simulink model "S1_ContinuousDCMotorSimulationSampled"  (R2018b)
settings: Solver=VariableStepAuto  StartTime=0.0  StopTime=25  MaxStep=Ts  RelTol=1e-3
undefined symbols (not defined in the file): C0, DiscIntNeverNeededParam, F, Imax, Imin, J, Ke, Km, Kphi, L, R, Ts, TsMeca, Vmax, Vmin
libraries: simulink x7
Description:
  | Continuous time model of the DC motor
  | 
  | Cascaded speed control :
  | - Inner loop : electrical control (state feedback with integral action)
  | - Outer loop :  mechanical control (state feedback with integral action)
  | - Clamping : Enable or disable integral actions
settings Model: Creator=R.Delpoux & L.Kerhuel  LastModifiedBy=rdelpoux
settings SolverCC: ZeroCrossControl=DisableAll
settings SFSimCC: SimUseLocalCustomCode=off
settings RTWCC: RTWUseLocalCustomCode=off

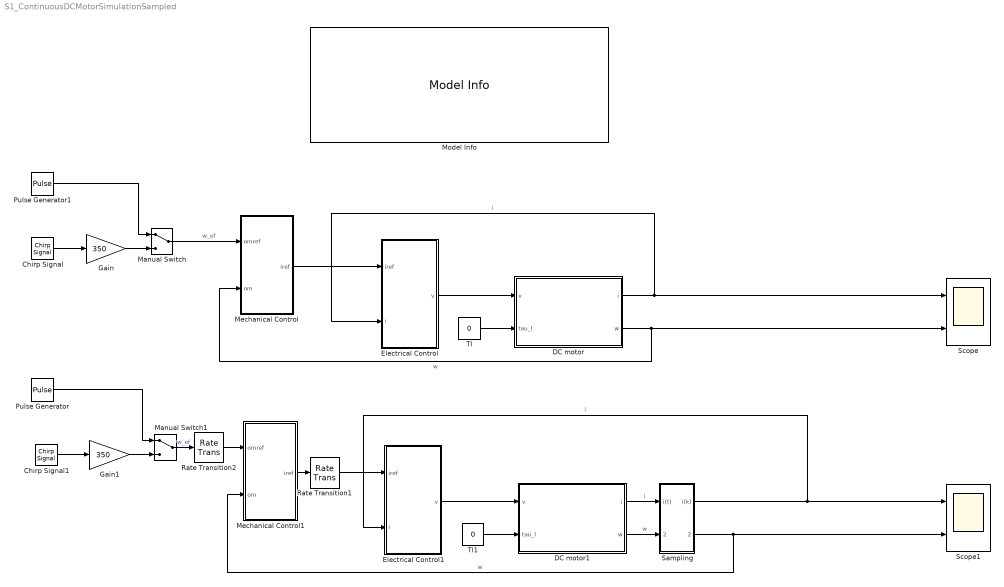
== system S1_ContinuousDCMotorSimulationSampled ==
  Chirp Signal : simulink/Sources/Chirp Signal  f1=0.1  T=20  f2=5
  Chirp Signal1 : simulink/Sources/Chirp Signal  f1=0.1  T=20  f2=5
  DC motor : Subsystem  mask(Motor PRAVALUX MPM4-0002){R=R, L=L, Kphi=Kphi, J=J, F=F, C0=C0}
      mask prompts: R "Resistance (R) in Ohms"; L "Inductance (L) in H"; Kphi "Back EMF (Kphi) in V/rad/s"; J "J in kgm²"; F "F in N/rad/s"
      mask help:
      | Continuous time Model for PRAVALUX MPM4 DC motor
      | Caracteristics: 24V DC, 90W, 5.2A, 3000RPM
      |
      | It is a 2nd order model made of two intertwinned system:
      | one 1st order electrical system and one 1st order mechanical system.
      |
      | Look under mask (Ctrl-U) to see the model
      mask DialogControl Container11 Prompt: Motor
      mask DialogControl Container3 Prompt: Electrical Parameters
      mask DialogControl Container3_copy Prompt: Mechanical Parameters
      mask Display:
      | color('green');
      | image('MotorPravalux.png');
      | %port_label('input',1,'DC');
      | %port_label('output',1,'BEMF');
  DC motor1 : Subsystem  mask(Motor PRAVALUX MPM4-0002){R=R, L=L, Kphi=Kphi, J=J, F=F, C0=C0}
      mask prompts: R "Resistance (R) in Ohms"; L "Inductance (L) in H"; Kphi "Back EMF (Kphi) in V/rad/s"; J "J in kgm²"; F "F in N/rad/s"
      mask help:
      | Continuous time Model for PRAVALUX MPM4 DC motor
      | Caracteristics: 24V DC, 90W, 5.2A, 3000RPM
      |
      | It is a 2nd order model made of two intertwinned system:
      | one 1st order electrical system and one 1st order mechanical system.
      |
      | Look under mask (Ctrl-U) to see the model
      mask DialogControl Container11 Prompt: Motor
      mask DialogControl Container3 Prompt: Electrical Parameters
      mask DialogControl Container3_copy Prompt: Mechanical Parameters
      mask Display:
      | color('green');
      | image('MotorPravalux.png');
      | %port_label('input',1,'DC');
      | %port_label('output',1,'BEMF');
  Electrical Control : Subsystem
  Electrical Control1 : Subsystem
  Gain : Gain  Gain=350  OutDataTypeStr=Inherit: Inherit via back propagation
  Gain1 : Gain  Gain=350  OutDataTypeStr=Inherit: Inherit via back propagation
  Manual Switch : ManualSwitch
  Manual Switch1 : ManualSwitch
  Mechanical Control : Subsystem
  Mechanical Control1 : Subsystem
  Model Info : simulink/Model-Wide Utilities/Model Info  Frame=on  DisplayStringWithTags=|  HorizontalTextAlignment=Center  LeftAlignmentValue=0.5
      | %<ModelName> v%<ModelVersion> - %<Creator>
      | 
      | %<Description>
      | 
      | Lost modified on: %<LastModificationDate>
  Pulse Generator : DiscretePulseGenerator  PulseType=Time based  Amplitude=200  PulseWidth=50  PhaseDelay=0.5  SampleTime=-1
  Pulse Generator1 : DiscretePulseGenerator  PulseType=Time based  Amplitude=200  PulseWidth=50  PhaseDelay=0.5  SampleTime=-1
  Rate Transition1 : RateTransition  Deterministic=off
  Rate Transition2 : RateTransition  Deterministic=off
  Sampling : Subsystem
  Scope : Scope  NumInputPorts=2
  Scope1 : Scope  NumInputPorts=2
  Tl : Constant  Value=0
  Tl1 : Constant  Value=0
  wires:
  Electrical Control/1(v) -> DC motor/1(v)
  DC motor/1(i) -> Electrical Control/2(i), Scope/1  "i"
  DC motor/2(w) -> Scope/2, Mechanical Control/2(om)  "w"
  Manual Switch/1 -> Mechanical Control/1(omref)  "w_ef"
  Mechanical Control/1(iref) -> Electrical Control/1(iref)
  Tl/1 -> DC motor/2(tau_l)
  Gain/1 -> Manual Switch/2
  Chirp Signal/1 -> Gain/1
  Pulse Generator1/1 -> Manual Switch/1
  Pulse Generator/1 -> Manual Switch1/1
  Electrical Control1/1(v) -> DC motor1/1(v)
  Tl1/1 -> DC motor1/2(tau_l)
  Gain1/1 -> Manual Switch1/2
  Chirp Signal1/1 -> Gain1/1
  Manual Switch1/1 -> Rate Transition2/1  "w_ef"
  DC motor1/1(i) -> Sampling/1(i(t))  "i"
  DC motor1/2(w) -> Sampling/2(w(t))  "w"
  Sampling/1(i(k)) -> Electrical Control1/2(i), Scope1/1  "i"
  Sampling/2(w(k)) -> Scope1/2, Mechanical Control1/2(om)  "w"
  Mechanical Control1/1(iref) -> Rate Transition1/1
  Rate Transition1/1 -> Electrical Control1/1(iref)
  Rate Transition2/1 -> Mechanical Control1/1(omref)

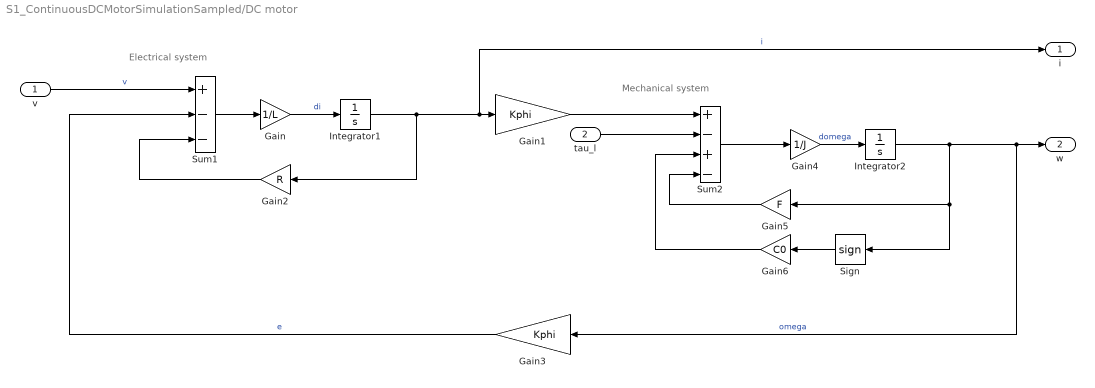
== system S1_ContinuousDCMotorSimulationSampled/DC motor ==
  note: Mechanical system
  note: Electrical system
  v : Inport  SampleTime=0
  tau_l : Inport  Port=2
  Gain : Gain  Gain=1/L
  Gain1 : Gain  Gain=Kphi
  Gain2 : Gain  Gain=R
  "Gain3  " : Gain  Gain=Kphi
  Gain4 : Gain  Gain=1/J
  Gain5 : Gain  Gain=F
  Gain6 : Gain  Gain=C0
  Integrator1 : Integrator
  Integrator2 : Integrator
  Sign : Signum
  Sum1 : Sum  Inputs=+--
  Sum2 : Sum  Inputs=+-+-
  i : Outport
  w : Outport  Port=2
  wires:
  Sum1/1 -> Gain/1
  Gain/1 -> Integrator1/1  "di"
  Integrator1/1 -> Gain2/1, i/1, Gain1/1  "i"
  v/1 -> Sum1/1  "v"
  Gain2/1 -> Sum1/3
  "Gain3  "/1 -> Sum1/2  "e"
  tau_l/1 -> Sum2/2
  Gain6/1 -> Sum2/3
  Sign/1 -> Gain6/1
  Integrator2/1 -> "Gain3  "/1, w/1, Sign/1, Gain5/1  "omega"
  Gain5/1 -> Sum2/4
  Sum2/1 -> Gain4/1
  Gain4/1 -> Integrator2/1  "domega"
  Gain1/1 -> Sum2/1

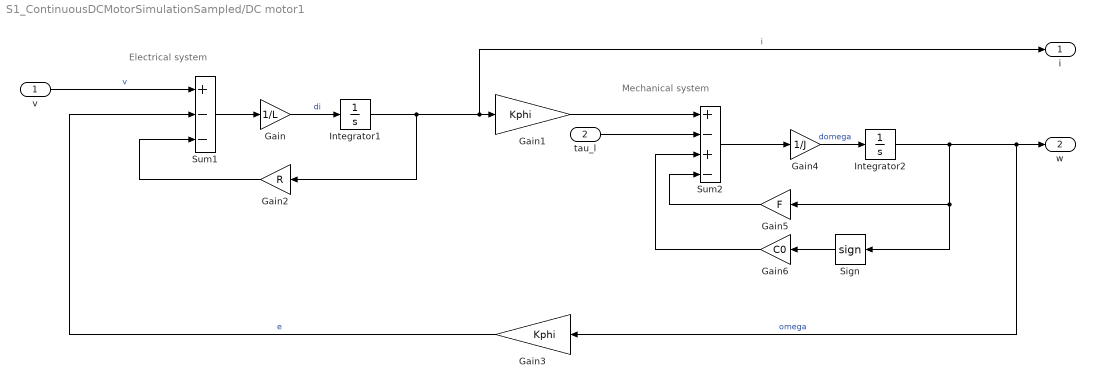
== system S1_ContinuousDCMotorSimulationSampled/DC motor1 ==
  note: Mechanical system
  note: Electrical system
  v : Inport  SampleTime=0
  tau_l : Inport  Port=2
  Gain : Gain  Gain=1/L
  Gain1 : Gain  Gain=Kphi
  Gain2 : Gain  Gain=R
  "Gain3  " : Gain  Gain=Kphi
  Gain4 : Gain  Gain=1/J
  Gain5 : Gain  Gain=F
  Gain6 : Gain  Gain=C0
  Integrator1 : Integrator
  Integrator2 : Integrator
  Sign : Signum
  Sum1 : Sum  Inputs=+--
  Sum2 : Sum  Inputs=+-+-
  i : Outport
  w : Outport  Port=2
  wires:
  Sum1/1 -> Gain/1
  Gain/1 -> Integrator1/1  "di"
  Integrator1/1 -> Gain2/1, i/1, Gain1/1  "i"
  v/1 -> Sum1/1  "v"
  Gain2/1 -> Sum1/3
  "Gain3  "/1 -> Sum1/2  "e"
  tau_l/1 -> Sum2/2
  Gain6/1 -> Sum2/3
  Sign/1 -> Gain6/1
  Integrator2/1 -> "Gain3  "/1, w/1, Sign/1, Gain5/1  "omega"
  Gain5/1 -> Sum2/4
  Sum2/1 -> Gain4/1
  Gain4/1 -> Integrator2/1  "domega"
  Gain1/1 -> Sum2/1

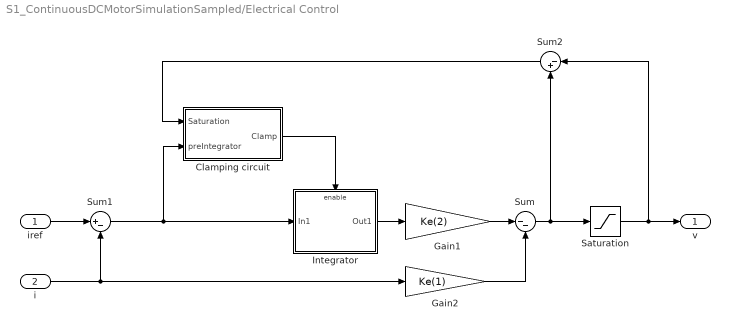
== system S1_ContinuousDCMotorSimulationSampled/Electrical Control ==
  iref : Inport
  i : Inport  Port=2
  Clamping circuit : Subsystem
  Gain1 : Gain  Gain=Ke(2)
  Gain2 : Gain  Gain=Ke(1)
  Integrator : Subsystem
  Saturation : Saturate  UpperLimit=Vmax  LowerLimit=Vmin
  Sum : Sum  Inputs=|--
  Sum1 : Sum  Inputs=|+-
  Sum2 : Sum  Inputs=|-+  OutDataTypeStr=Inherit: Same as accumulator
  v : Outport
  wires:
  iref/1 -> Sum1/1
  i/1 -> Gain2/1, Sum1/2
  Gain1/1 -> Sum/1
  Gain2/1 -> Sum/2
  Saturation/1 -> Sum2/1, v/1
  Sum1/1 -> Integrator/1(In1), Clamping circuit/2(preIntegrator)
  Integrator/1(Out1) -> Gain1/1
  Clamping circuit/1(Clamp) -> Integrator/Enable
  Sum/1 -> Saturation/1, Sum2/2
  Sum2/1 -> Clamping circuit/1(Saturation)

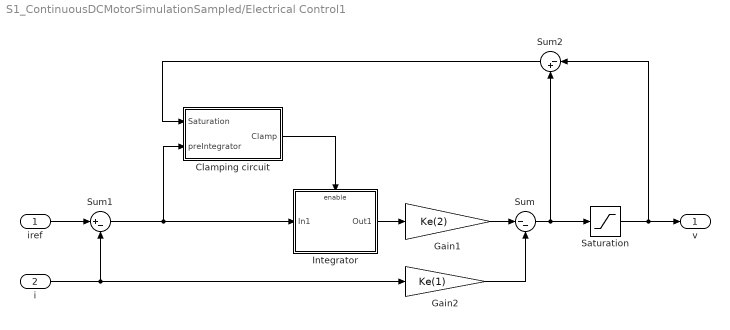
== system S1_ContinuousDCMotorSimulationSampled/Electrical Control1 ==
  iref : Inport
  i : Inport  Port=2
  Clamping circuit : Subsystem
  Gain1 : Gain  Gain=Ke(2)
  Gain2 : Gain  Gain=Ke(1)
  Integrator : Subsystem
  Saturation : Saturate  UpperLimit=Vmax  LowerLimit=Vmin
  Sum : Sum  Inputs=|--
  Sum1 : Sum  Inputs=|+-
  Sum2 : Sum  Inputs=|-+  OutDataTypeStr=Inherit: Same as accumulator
  v : Outport
  wires:
  iref/1 -> Sum1/1
  i/1 -> Gain2/1, Sum1/2
  Gain1/1 -> Sum/1
  Gain2/1 -> Sum/2
  Saturation/1 -> Sum2/1, v/1
  Sum1/1 -> Integrator/1(In1), Clamping circuit/2(preIntegrator)
  Integrator/1(Out1) -> Gain1/1
  Clamping circuit/1(Clamp) -> Integrator/Enable
  Sum/1 -> Saturation/1, Sum2/2
  Sum2/1 -> Clamping circuit/1(Saturation)

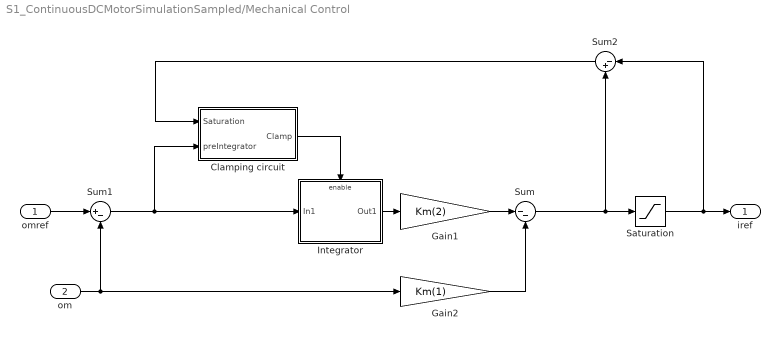
== system S1_ContinuousDCMotorSimulationSampled/Mechanical Control ==
  omref : Inport
  om : Inport  Port=2
  Clamping circuit : Subsystem
  Gain1 : Gain  Gain=Km(2)
  Gain2 : Gain  Gain=Km(1)
  Integrator : Subsystem
  Saturation : Saturate  UpperLimit=Imax  LowerLimit=Imin
  Sum : Sum  Inputs=|--
  Sum1 : Sum  Inputs=|+-
  Sum2 : Sum  Inputs=|-+  OutDataTypeStr=Inherit: Same as accumulator
  iref : Outport
  wires:
  Gain1/1 -> Sum/1
  Sum1/1 -> Clamping circuit/2(preIntegrator), Integrator/1(In1)
  omref/1 -> Sum1/1
  Gain2/1 -> Sum/2
  om/1 -> Gain2/1, Sum1/2
  Sum2/1 -> Clamping circuit/1(Saturation)
  Sum/1 -> Sum2/2, Saturation/1
  Clamping circuit/1(Clamp) -> Integrator/Enable
  Saturation/1 -> Sum2/1, iref/1
  Integrator/1(Out1) -> Gain1/1

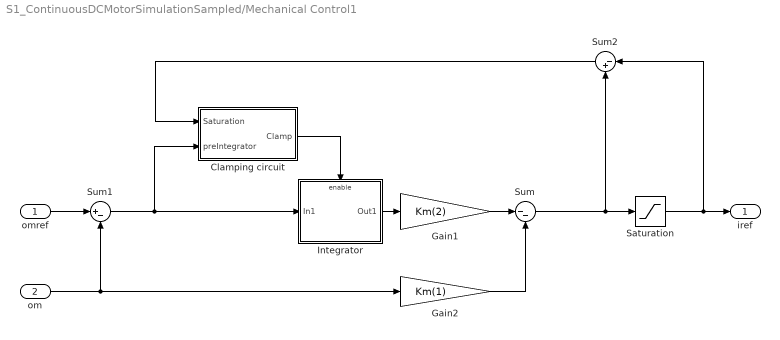
== system S1_ContinuousDCMotorSimulationSampled/Mechanical Control1 ==
  omref : Inport
  om : Inport  Port=2
  Clamping circuit : Subsystem
  Gain1 : Gain  Gain=Km(2)
  Gain2 : Gain  Gain=Km(1)
  Integrator : Subsystem
  Saturation : Saturate  UpperLimit=Imax  LowerLimit=Imin
  Sum : Sum  Inputs=|--
  Sum1 : Sum  Inputs=|+-
  Sum2 : Sum  Inputs=|-+  OutDataTypeStr=Inherit: Same as accumulator
  iref : Outport
  wires:
  Gain1/1 -> Sum/1
  Sum1/1 -> Clamping circuit/2(preIntegrator), Integrator/1(In1)
  omref/1 -> Sum1/1
  Gain2/1 -> Sum/2
  om/1 -> Gain2/1, Sum1/2
  Sum2/1 -> Clamping circuit/1(Saturation)
  Sum/1 -> Sum2/2, Saturation/1
  Clamping circuit/1(Clamp) -> Integrator/Enable
  Saturation/1 -> Sum2/1, iref/1
  Integrator/1(Out1) -> Gain1/1

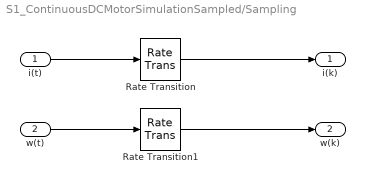
== system S1_ContinuousDCMotorSimulationSampled/Sampling ==
  i(t) : Inport
  w(t) : Inport  Port=2
  Rate Transition : RateTransition  Deterministic=off  OutPortSampleTime=Ts
  Rate Transition1 : RateTransition  Deterministic=off  OutPortSampleTime=TsMeca
  i(k) : Outport
  w(k) : Outport  Port=2
  wires:
  Rate Transition/1 -> i(k)/1
  i(t)/1 -> Rate Transition/1
  w(t)/1 -> Rate Transition1/1
  Rate Transition1/1 -> w(k)/1

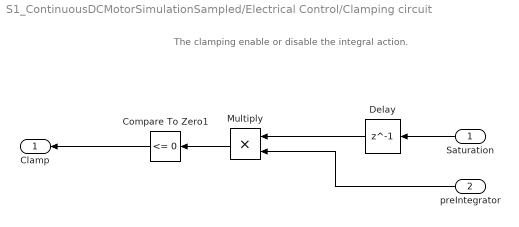
== system S1_ContinuousDCMotorSimulationSampled/Electrical Control/Clamping circuit ==
  note: The clamping enable or disable the integral action.
  Saturation : Inport  DisableCoverage=on
  preIntegrator : Inport  DisableCoverage=on  Port=2
  Compare To Zero1 : simulink/Logic and Bit Operations/Compare To Zero  relop=<=  OutDataTypeStr=boolean
  Delay : Delay  DelayLength=1  InitialCondition=0
  Multiply : Product
  Clamp : Outport  DisableCoverage=on
  wires:
  Compare To Zero1/1 -> Clamp/1
  preIntegrator/1 -> Multiply/2
  Multiply/1 -> Compare To Zero1/1
  Saturation/1 -> Delay/1
  Delay/1 -> Multiply/1

== system S1_ContinuousDCMotorSimulationSampled/Electrical Control/Integrator ==
  In1 : Inport
  Enable : EnablePort
  Integrator : Integrator
  Out1 : Outport
  wires:
  Integrator/1 -> Out1/1
  In1/1 -> Integrator/1

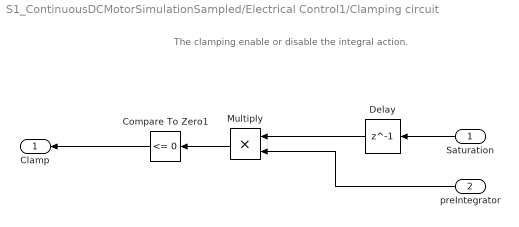
== system S1_ContinuousDCMotorSimulationSampled/Electrical Control1/Clamping circuit ==
  note: The clamping enable or disable the integral action.
  Saturation : Inport  DisableCoverage=on
  preIntegrator : Inport  DisableCoverage=on  Port=2
  Compare To Zero1 : simulink/Logic and Bit Operations/Compare To Zero  relop=<=  OutDataTypeStr=boolean
  Delay : Delay  DelayLength=1  InitialCondition=0
  Multiply : Product
  Clamp : Outport  DisableCoverage=on
  wires:
  Compare To Zero1/1 -> Clamp/1
  preIntegrator/1 -> Multiply/2
  Multiply/1 -> Compare To Zero1/1
  Saturation/1 -> Delay/1
  Delay/1 -> Multiply/1

== system S1_ContinuousDCMotorSimulationSampled/Electrical Control1/Integrator ==
  In1 : Inport
  Enable : EnablePort
  Discrete-Time Integrator : DiscreteIntegrator  SampleTime=Ts  ICPrevOutput=DiscIntNeverNeededParam  ICPrevScaledInput=DiscIntNeverNeededParam
  Out1 : Outport
  wires:
  Discrete-Time Integrator/1 -> Out1/1
  In1/1 -> Discrete-Time Integrator/1

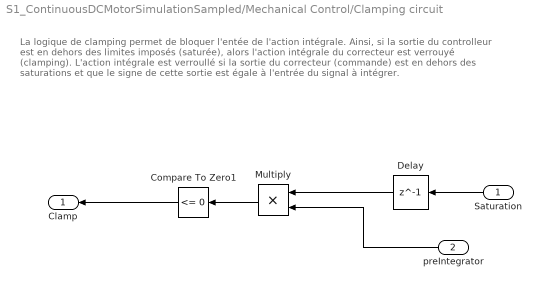
== system S1_ContinuousDCMotorSimulationSampled/Mechanical Control/Clamping circuit ==
  note: La logique de clamping permet de bloquer l'entée de l'action intégrale.
      | Ainsi, si la sortie du controlleur est en dehors des limites imposés (saturée), alors l'action intégrale du correcteur est verrouyé (clamping).
      | L'action intégrale est verroullé si la sortie du correcteur (commande) est en dehors des saturations et que le signe de cette sortie est égale
      | à l'entrée du signal à intégrer.
  Saturation : Inport  DisableCoverage=on
  preIntegrator : Inport  DisableCoverage=on  Port=2
  Compare To Zero1 : simulink/Logic and Bit Operations/Compare To Zero  relop=<=  OutDataTypeStr=boolean
  Delay : Delay  DelayLength=1  InitialCondition=0
  Multiply : Product
  Clamp : Outport  DisableCoverage=on
  wires:
  Compare To Zero1/1 -> Clamp/1
  preIntegrator/1 -> Multiply/2
  Multiply/1 -> Compare To Zero1/1
  Saturation/1 -> Delay/1
  Delay/1 -> Multiply/1

== system S1_ContinuousDCMotorSimulationSampled/Mechanical Control/Integrator ==
  In1 : Inport
  Enable : EnablePort
  Integrator : Integrator
  Out1 : Outport
  wires:
  Integrator/1 -> Out1/1
  In1/1 -> Integrator/1

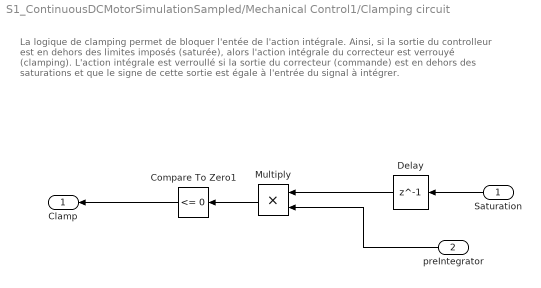
== system S1_ContinuousDCMotorSimulationSampled/Mechanical Control1/Clamping circuit ==
  note: La logique de clamping permet de bloquer l'entée de l'action intégrale.
      | Ainsi, si la sortie du controlleur est en dehors des limites imposés (saturée), alors l'action intégrale du correcteur est verrouyé (clamping).
      | L'action intégrale est verroullé si la sortie du correcteur (commande) est en dehors des saturations et que le signe de cette sortie est égale
      | à l'entrée du signal à intégrer.
  Saturation : Inport  DisableCoverage=on
  preIntegrator : Inport  DisableCoverage=on  Port=2
  Compare To Zero1 : simulink/Logic and Bit Operations/Compare To Zero  relop=<=  OutDataTypeStr=boolean
  Delay : Delay  DelayLength=1  InitialCondition=0
  Multiply : Product
  Clamp : Outport  DisableCoverage=on
  wires:
  Compare To Zero1/1 -> Clamp/1
  preIntegrator/1 -> Multiply/2
  Multiply/1 -> Compare To Zero1/1
  Saturation/1 -> Delay/1
  Delay/1 -> Multiply/1

== system S1_ContinuousDCMotorSimulationSampled/Mechanical Control1/Integrator ==
  In1 : Inport
  Enable : EnablePort
  Discrete-Time Integrator : DiscreteIntegrator  SampleTime=TsMeca  ICPrevOutput=DiscIntNeverNeededParam  ICPrevScaledInput=DiscIntNeverNeededParam
  Out1 : Outport
  wires:
  Discrete-Time Integrator/1 -> Out1/1
  In1/1 -> Discrete-Time Integrator/1
